simulink model "sin_to_mod1"  (Simulink 8.1)
settings: Solver=ode3  StartTime=0.0  StopTime=0.1  RelTol=1e-3
undefined symbols (not defined in the file): Fs, modctrl, OSR, sinamp, sinfreq
libraries: dspsigops x2, dspsrcs4 x2, dsparch4 x1
settings Model: Creator=amyles  LastModifiedBy=amyles
settings DataIOCC: LimitDataPoints=off  MaxDataPoints=50000
settings DebuggingCC: StrictBusMsg=Warning

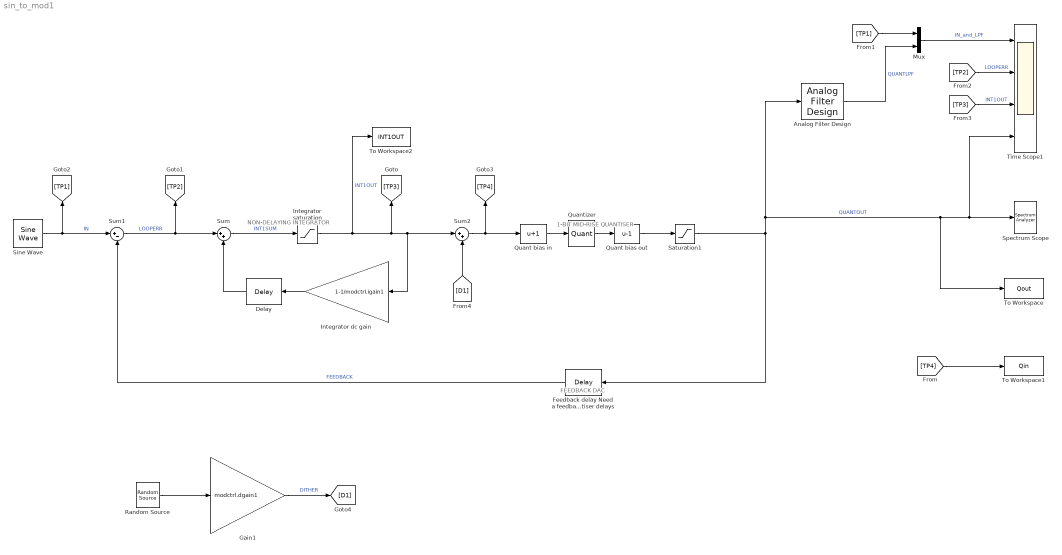
== system sin_to_mod1 ==
  note: 1-BIT MID-RISE QUANTISER
  note: NON-DELAYING INTEGRATOR
  note: FEEDBACK DAC
  Analog Filter Design : dsparch4/Analog Filter Design  method=Butterworth  filttype=Lowpass  N=8  Wlo=pi*Fs/OSR  Whi=80  Rp=2  Rs=40
      settings: AttributesFormatString=Low-pass filter the loop output\nto illustrate intuitively how the\npulse density modulated +1/-1\noutput stream does indeed capture\nthe input signal
  Delay : dspsigops/Delay  InputProcessing=Columns as channels (frame based)  dly_unit=Samples  delay=1  ic_detail=off  dif_ic_for_ch=off  dif_ic_for_dly=off  ic=0  reset_popup=None
  Feedback delay Need a feedback delay to avoid a delay-free loop as we have no integrator or quantiser delays : dspsigops/Delay  InputProcessing=Columns as channels (frame based)  dly_unit=Samples  delay=1  ic_detail=off  dif_ic_for_ch=off  dif_ic_for_dly=off  ic=0  reset_popup=None
  Gain1 : Gain  Gain=modctrl.dgain1
      settings: AttributesFormatString=Dither level adjust
  Integrator dc gain : Gain  Gain=1-1/modctrl.igain1
      settings: AttributesFormatString=Integrator leakage\n(model finite integrator dc/LF\ngain in analog modulators)
  Integrator saturation : Saturate  UpperLimit=modctrl.isat1  LowerLimit=-(modctrl.isat1)
      settings: AttributesFormatString=Real integrators will have\noutput swing limits (analog\nsignal headroom or digital\naccumulator min/max values.)
  Mux : Mux  Inputs=2
  Quant bias in : Bias  Bias=1
      settings: AttributesFormatString=Need offset to give\nMID-RISE quantiser
  Quant bias out : Bias  Bias=-1
      settings: AttributesFormatString=Shift outputs to\n..., -2, 1, 1, ...
  Quantizer : Quantizer  QuantizationInterval=2  LinearizeAsGain=off
      settings: AttributesFormatString=step = 2
  Random Source : dspsrcs4/Random Source  SrcType=Uniform  NormMethod=Ziggurat  CltLength=12  MinVal=-1  MaxVal=1  MeanVal=0  VarVal=1  RepMode=Not repeatable  rawSeed=1  IsInherit=off  SampMode=Discrete  SampTime=1/Fs  SampFrame=1  DataType=Double  OutComplex=Real
      settings: AttributesFormatString=Dither source
  Saturation1 : Saturate  UpperLimit=1  LowerLimit=-1
      settings: AttributesFormatString=Limit quantiser\noutput to +/-1
  Sine Wave : dspsrcs4/Sine Wave  Amplitude=sinamp  Frequency=sinfreq  Phase=0  SampleMode=Discrete  OutComplex=Real  CompMethod=Trigonometric fcn  TableSize=Speed  SampleTime=1/Fs  SamplesPerFrame=1  ResetState=Restart at time zero  dataType=double  wordLen=16  udDataType=sfix(16)  fracBitsMode=Best precision  numFracBits=15  OutDataTypeStr=double  LastOutDataTypeStr=double
  Spectrum Scope : SpectrumAnalyzer
      settings: CopyFcn=scopeextensions.ScopeBlock.callback(gcbh, 'onBlockCopy', gcbh);  DeleteFcn=scopeextensions.ScopeBlock.callback(gcbh, 'onBlockDelete');  PreSaveFcn=scopeextensions.ScopeBlock.callback(gcbh, 'onModelSave');  NameChangeFcn=scopeextensions.ScopeBlock.callback(gcbh, 'onBlockRename');  CloseFcn=scopeextensions.ScopeBlock.callback(gcbh, 'onBlockClose');  PreDeleteFcn=scopeextensions.ScopeBlock.callback(gcbh, 'onBlockPreDelete');
  Sum : Sum  Inputs=|++
      settings: AttributesFormatString=Integrator summer
  Sum1 : Sum  Inputs=|+-
      settings: AttributesFormatString=Modulator input\nloop servo error (input - fbk)
  Sum2 : Sum  Inputs=|++
  Time Scope1 : Scope  NumInputPorts=4
      settings: TimeRange=0.01  YMin=-5~-1.2~-2.5~-1.2  YMax=5~1.2~2.5~1.2  DataFormat=Structure  MaxDataPoints=10000
  To Workspace : ToWorkspace  VariableName=Qout  SampleTime=-1
      settings: AttributesFormatString=Export SDM output\nto workspace for\npost-processing
  To Workspace1 : ToWorkspace  VariableName=Qin  SampleTime=-1
      settings: AttributesFormatString=Export Quant' input\nto workspace for\npost-processing\n(e.g quantiser gain)
  To Workspace2 : ToWorkspace  VariableName=INT1OUT  SampleTime=-1
  wires:
  Delay/1 -> Sum/2
  Sum/1 -> Integrator saturation/1  "INT1SUM"
  Sum1/1 -> Sum/1, [TP2]  "LOOPERR"
  Feedback delay Need a feedback delay to avoid a delay-free loop as we have no integrator or quantiser delays/1 -> Sum1/2  "FEEDBACK"
  Sine Wave/1 -> Sum1/1, [TP1]  "IN"
  Analog Filter Design/1 -> Mux/2  "QUANTLPF"
  Sum2/1 -> [TP4], Quant bias in/1
  Random Source/1 -> Gain1/1
  Integrator dc gain/1 -> Delay/1
  Saturation1/1 -> Analog Filter Design/1, To Workspace/1, Spectrum Scope/1, Time Scope1/4, Feedback delay Need a feedback delay to avoid a delay-free loop as we have no integrator or quantiser delays/1  "QUANTOUT"
  Quant bias out/1 -> Saturation1/1
  Integrator saturation/1 -> Sum2/1, Integrator dc gain/1, [TP3], To Workspace2/1  "INT1OUT"
  Mux/1 -> Time Scope1/1  "IN_and_LPF"
  [TP4] -> To Workspace1/1
  [TP1] -> Mux/1
  [TP2] -> Time Scope1/2  "LOOPERR"
  [TP3] -> Time Scope1/3  "INT1OUT"
  Gain1/1 -> [D1]  "DITHER"
  [D1] -> Sum2/2
  Quant bias in/1 -> Quantizer/1
  Quantizer/1 -> Quant bias out/1
